simulink library "FadeBtc"  (R2022b)
settings: Solver=VariableStepAuto  StartTime=0.0  StopTime=10.0  RelTol=1e-3
libraries: HandyTextFile x2, FadeControlBtc x1, FadeRamperBtc x1
settings Model: Creator=st51187  LastModifiedBy=kl13806
settings SolverCC: AlgebraicLoopSolver=TrustRegion
settings DebuggingCC: UnconnectedInputMsg=warning  UnconnectedOutputMsg=warning  UnconnectedLineMsg=warning  SFMachineParentedDataDiag=warning
settings ModelReferenceCC: EnableRefExpFcnMdlSchedulingChecks=on
settings RTWCC: DLArmComputeVersion=19.05

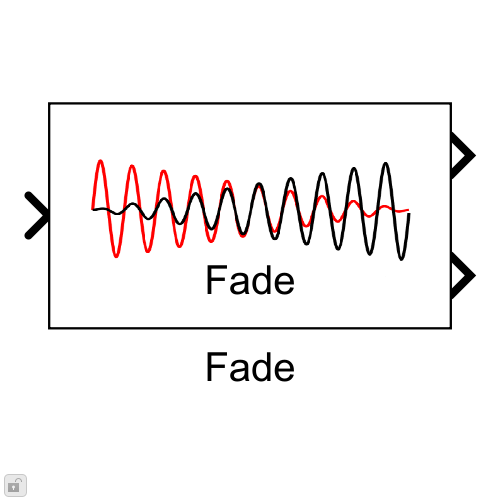
[thumbnail: Simulink's stored preview of the top-level diagram]
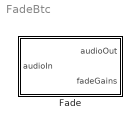
== system FadeBtc ==
  Fade : Subsystem  mask(Blocklib Fade){Config=[], FeatureName=Fade, EnableGainOut=on}
      mask prompts: Config "FadeConfig"; FeatureName "Feature path name:"; EnableGainOut "Enable output gain port"
      mask help: This block groups its input channels as 'Front' and 'Rear' and applies a fade forward or backward effect by using a combination of low pass and high pass filters.
      mask init:
      | blkh=gcbh;
      | Config=BTConfig.Assert(blkh,Config);
      | BTConfig.InitSetFeatureIfPresent(blkh,'FeatureName');
      | Config.Validate();
      | 
      | % Mask Init code
      | EnableBlockPort(blkh,'fadeGains',EnableGainOut);
      mask Help:
      | The Fade block includes runtime control support for adjusting the fade dynamically.
      | MASK PARAMETERS
      | - The Index offset determines the index which corresponds to the fade being in the center position (typically 128).
      | - Channels may to be assigned to either the Front ('1') or Rear ('2') groups. This field is set up as an array of channels with every channel assigned to atleast one valid group.
      | - 'Enable silent extreme' mutes the speakers of the group whose gains are being 'cut' when at extreme indices.
      | - 'Disable boost' determines whether a boost is required or not. If selected, the maximum boost will be '1' on the linear scale ('0' in dB), otherwise it is computed from the 'cut' gains (typically a maximum of 3 dB).
      | 
      | OUTPUTS
      | - audioOut
      | - fadeGains : 1x2 array [frontGain, rearGain]
      | 
      | RTC
      | Control messages can be sent through the RTC block. The block is configured to accept an index which determines the gains for each channel group, a ramp rate or time (the rate has precedence).
      | E.g., RTC_SIM_OBJ.AddREQ( 'FadeSet', 0.1, [0001, <fade_index>, <ramp_db_per_second>, <ramp_milliseconds>]);
      mask Callback Config: BTConfig.CallbackHideIfPresent(gcbh,{'FeatureName'});
      mask TypeOptions FeatureName: FadeControl/FeatureName | FadeRamper/FeatureName
      mask DialogControl ParameterText1 Prompt: The following operations are available to control the behavior of the block.
      mask DialogControl ParameterText3 Prompt: 'Index Scale' determines the total fade levels, while 'Index Offset' determines the index at which no fade is applied to the input audio. Input channels are to be mapped to either the 'Front' (1) or 'Rear' (2) channel groups. Enabling 'Silent extreme' mutes the speakers belonging to the opposite group, when the audio is faded completely forward or backward. 'Disable boost' sets the boost to 0 dB.
      mask Display:
      | image('Fade.png');
      | 
      | % retrieve the block's pixel size
      | pos = get(gcbh,'position');
      | bw = pos(3) - pos(1);
      | bh = pos(4) - pos(2);
      | 
      | % place feature name text
      | text(bw*0.5, 0, [FeatureName '\n\n'], 'horizontalAlignment', 'center');

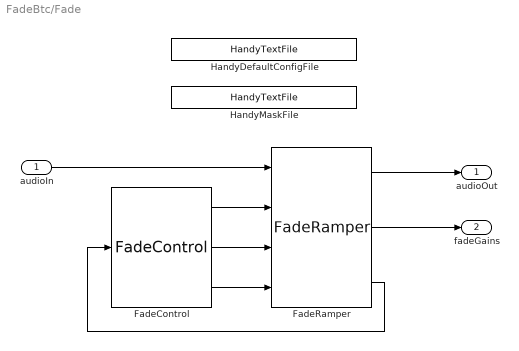
== system FadeBtc/Fade ==
  audioIn : Inport
  FadeControl : FadeControlBtc/FadeControl  Config=Config  FeatureName=Fade
      settings: SourceProductName=Bose Blocklib
  FadeRamper : FadeRamperBtc/FadeRamper  Config=Config  FeatureName=Fade  EnableGainOut=on
      settings: SourceProductName=Bose Blocklib
  HandyDefaultConfigFile : HandyTextFile/HandyTextFile  TemplateSource=Config  FileSuffix=Init  OpenDialogOnLoad=off  UseThisBlockName=off  TheDefaultText=|  ShowInLibBrowser=on
      | % $(FILENAME) Setup model parameters for each "Init" callback (e.g. update diagram)
      | sample_rate_in_hertz = 44100;
      | frame_size = 32;
      | sysin_channel_count = 2;
  HandyMaskFile : HandyTextFile/HandyTextFile  TemplateSource=Mask  FileSuffix=Init  OpenDialogOnLoad=off  UseThisBlockName=off  TheDefaultText=|  ShowInLibBrowser=on
      | % $(FILENAME) Setup model parameters for each "Init" callback (e.g. update diagram)
      | sample_rate_in_hertz = 44100;
      | frame_size = 32;
      | sysin_channel_count = 2;
  audioOut : Outport  VectorParamsAs1DForOutWhenUnconnected=off
  fadeGains : Outport  Port=2
  wires:
  FadeControl/1 -> FadeRamper/2
  FadeControl/2 -> FadeRamper/3
  FadeControl/3 -> FadeRamper/4
  audioIn/1 -> FadeRamper/1
  FadeRamper/3 -> FadeControl/1
  FadeRamper/1 -> audioOut/1
  FadeRamper/2 -> fadeGains/1
